simulink model "Quadrotor_Model_X"  (R2016a)
settings: Solver=VariableStepAuto  StartTime=0.0  StopTime=20  RelTol=1e-3
settings Model: Creator=SRQ  LastModifiedBy=SRQ

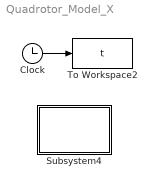
== system Quadrotor_Model_X ==
  Clock : Clock
  Subsystem4 : Subsystem
      mask Display: disp('X轴向与俯仰角');
  To Workspace2 : ToWorkspace  VariableName=t  SampleTime=-1
  wires:
  Clock/1 -> To Workspace2/1

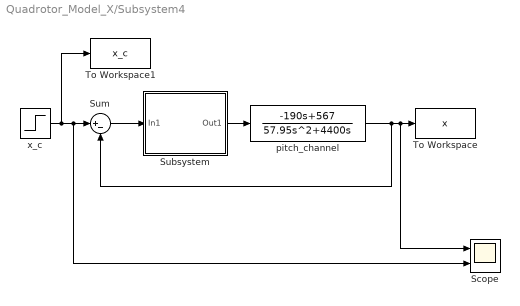
== system Quadrotor_Model_X/Subsystem4 ==
  Scope : Scope  NumInputPorts=2
  Subsystem : Subsystem  mask{kp=10, ki=0.1, kd=0.1}
      mask Display: disp('PID');
  Sum : Sum  Inputs=|+-
  To Workspace : ToWorkspace  VariableName=x  SampleTime=-1
  To Workspace1 : ToWorkspace  VariableName=x_c  SampleTime=-1
  pitch_channel : TransferFcn  Numerator=[-190 567]  Denominator=[57.95 4400 0]
  x_c : Step  Time=0  SampleTime=0
  wires:
  Sum/1 -> Subsystem/1(In1)
  Subsystem/1(Out1) -> pitch_channel/1
  pitch_channel/1 -> Sum/2, Scope/1, To Workspace/1
  x_c/1 -> To Workspace1/1, Scope/2, Sum/1

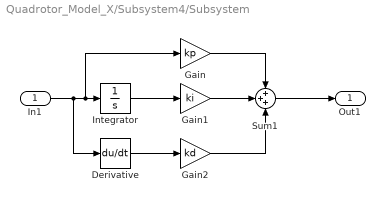
== system Quadrotor_Model_X/Subsystem4/Subsystem ==
  In1 : Inport
  Derivative : Derivative
  Gain : Gain  Gain=kp
  Gain1 : Gain  Gain=ki
  Gain2 : Gain  Gain=kd
  Integrator : Integrator
  Sum1 : Sum  Inputs=+++
  Out1 : Outport
  wires:
  Integrator/1 -> Gain1/1
  Derivative/1 -> Gain2/1
  Gain2/1 -> Sum1/3
  Gain/1 -> Sum1/1
  In1/1 -> Derivative/1, Gain/1, Integrator/1
  Sum1/1 -> Out1/1
  Gain1/1 -> Sum1/2
